simulink model "PresaDepredador_ejm1"  (R2020a)
settings: Solver=ode45  StartTime=0.0  StopTime=Time  RelTol=1e-3
undefined symbols (not defined in the file): alpha, beta, D0, delta, gamma, P0
settings Model: Creator=mluser  LastModifiedBy=curie
settings DataIOCC: SaveFormat=Array  ReturnWorkspaceOutputs=off

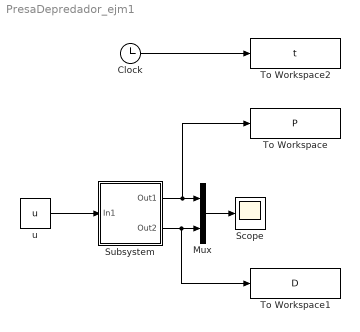
== system PresaDepredador_ejm1 ==
  Clock : Clock
  Mux : Mux  Inputs=2
  Scope : Scope
  Subsystem : Subsystem  mask{P0=P0, D0=D0, alpha=alpha, beta=beta, delta=delta, gamma=gamma}
      mask prompts: P0 "Condi. in. P"; alpha "tasa e crecimiento de P"
  To Workspace : ToWorkspace  VariableName=P  SampleTime=-1
      settings: Save2DSignal=2-D array (concatenate along first dimension)
  To Workspace1 : ToWorkspace  VariableName=D  SampleTime=-1
      settings: Save2DSignal=2-D array (concatenate along first dimension)
  To Workspace2 : ToWorkspace  VariableName=t  SampleTime=-1
      settings: Save2DSignal=2-D array (concatenate along first dimension)
  u : Constant  Value=u
  wires:
  Mux/1 -> Scope/1
  u/1 -> Subsystem/1(In1)
  Subsystem/1(Out1) -> To Workspace/1, Mux/1
  Subsystem/2(Out2) -> To Workspace1/1, Mux/2
  Clock/1 -> To Workspace2/1

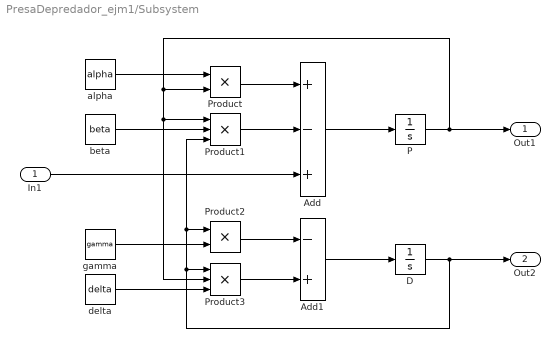
== system PresaDepredador_ejm1/Subsystem ==
  In1 : Inport
  Add : Sum  Inputs=+-+
  Add1 : Sum  Inputs=-+
  D : Integrator  InitialCondition=D0
  P : Integrator  InitialCondition=P0
  Product : Product
  Product1 : Product  Inputs=3
  Product2 : Product
  Product3 : Product  Inputs=3
  alpha : Constant  Value=alpha
  beta : Constant  Value=beta
  delta : Constant  Value=delta
  gamma : Constant  Value=gamma
  Out1 : Outport
  Out2 : Outport  Port=2
  wires:
  Product1/1 -> Add/2
  Add1/1 -> D/1
  alpha/1 -> Product/1
  D/1 -> Out2/1, Product1/3, Product2/1, Product3/1
  beta/1 -> Product1/2
  delta/1 -> Product3/3
  In1/1 -> Add/3
  P/1 -> Out1/1, Product3/2, Product1/1, Product/2
  Add/1 -> P/1
  gamma/1 -> Product2/2
  Product/1 -> Add/1
  Product3/1 -> Add1/2
  Product2/1 -> Add1/1
